simulink model "SHM_SIM"  (R2019b)
settings: Solver=ode23tb  StartTime=0.0  StopTime=T  MaxStep=1E-6  RelTol=1E-6
values from neighbouring files (symbols this model uses):
  f = 50    [SET_SIM.m]    (also in alphasolver.m = @(x) [(4/(pi))* VDC *(sin(x(1))-sin(x(2))+sin(x(3)))-V1)
  LL = 6.67e-3    (= 0.00667)    [SET_SIM.m]
  RL = 3.335    [SET_SIM.m]
  T_SMP = 2e-6    (= 2e-06)    [SET_SIM.m]
  VDC = 8.33    [SET_SIM.m]    (also in alphasolver.m = 24)
undefined symbols (not defined in the file or in its folder): a
libraries: powerlib x13, simulink x4, powerlib_meascontrol x2
settings Model: Creator=user  LastModifiedBy=ffara
settings DataIOCC: ReturnWorkspaceOutputs=off
settings DebuggingCC: ArithmeticOperatorsInVariantConditions=warning
settings SFSimCC: CustomCodeUndefinedFunction=UseInterfaceOnly

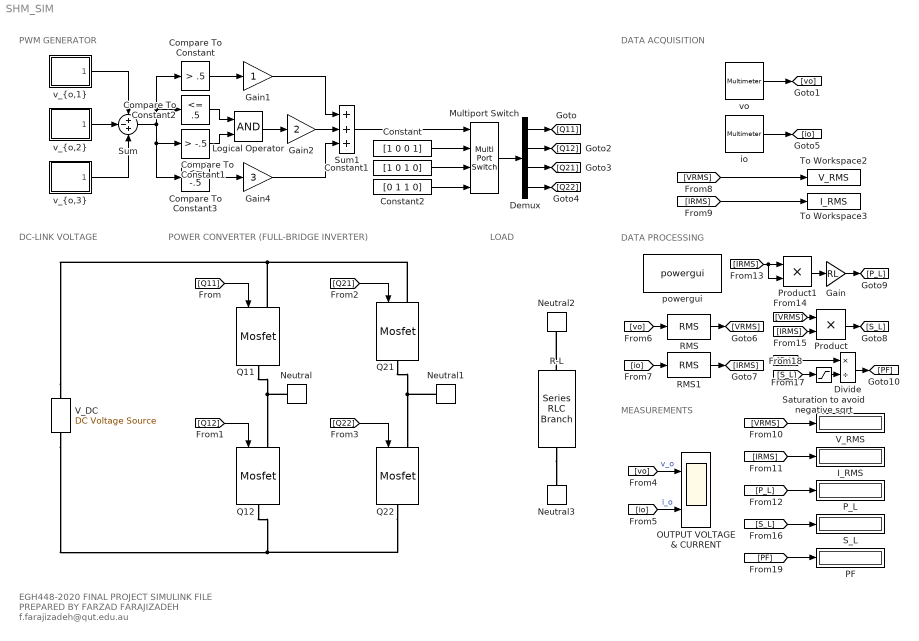
== system SHM_SIM ==
  note: EGH448-2020 FINAL PROJECT SIMULINK FILE
      | PREPARED BY FARZAD FARAJIZADEH
      | f.farajizadeh@qut.edu.au
  note: DATA ACQUISITION
  note: PWM GENERATOR
  note: LOAD
  note: POWER CONVERTER (FULL-BRIDGE INVERTER)
  note: DC-LINK VOLTAGE
  note: DATA PROCESSING
  note: MEASUREMENTS
  " OUTPUT VOLTAGE & CURRENT " : Scope  NumInputPorts=2
  Compare To Constant : simulink/Logic and Bit Operations/Compare To Constant  relop=>  const=.5  OutDataTypeStr=boolean
  Compare To Constant1 : simulink/Logic and Bit Operations/Compare To Constant  relop=>  const=-.5  OutDataTypeStr=boolean
  Compare To Constant2 : simulink/Logic and Bit Operations/Compare To Constant  relop=<=  const=.5  OutDataTypeStr=boolean
  Compare To Constant3 : simulink/Logic and Bit Operations/Compare To Constant  relop=<=  const=-.5  OutDataTypeStr=boolean
  Constant : Constant  Value=[1 0 0 1]
  Constant1 : Constant  Value=[1 0 1 0]
  Constant2 : Constant  Value=[0 1 1 0]
  Demux : Demux
  Divide : Product  Inputs=*/
  Gain : Gain  Gain=RL
  Gain1 : Gain
  Gain2 : Gain  Gain=2
  Gain4 : Gain  Gain=3
  I_RMS : Display
  Logical Operator : Logic  AllPortsSameDT=off  OutDataTypeStr=boolean
  Multiport Switch : MultiPortSwitch
  Neutral : powerlib/Elements/Neutral  LConnTagsString=a  NodeNumber=1
      settings: SourceProductName=Simscape Electrical  SourceProductBaseCode=PS
  Neutral1 : powerlib/Elements/Neutral  LConnTagsString=a  NodeNumber=2
      settings: SourceProductName=Simscape Electrical  SourceProductBaseCode=PS
  Neutral2 : powerlib/Elements/Neutral  LConnTagsString=a  NodeNumber=1
      settings: SourceProductName=Simscape Electrical  SourceProductBaseCode=PS
  Neutral3 : powerlib/Elements/Neutral  LConnTagsString=a  NodeNumber=2
      settings: SourceProductName=Simscape Electrical  SourceProductBaseCode=PS
  PF : Display
  P_L : Display
  Product : Product
  Product1 : Product
  Q{11..12,21..22} (4 alike) : powerlib/Power Electronics/Mosfet  Ron=0.001  Lon=0  Rd=0.001  Vfd=0  IC=0  Rs=1e5  Cs=inf  Measurements=off
      settings: SourceProductName=Simscape Electrical
  R-L : powerlib/Elements/Series RLC Branch  LConnTagsString=__new0  RConnTagsString=__new0  BranchType=RL  Resistance=RL  Inductance=LL  SetiL0=off  InitialCurrent=0  Capacitance=1e-6  Setx0=off  InitialVoltage=0  Measurements=Branch voltage and current
      settings: SourceProductName=Simscape Electrical
  RMS : powerlib_meascontrol/Measurements/RMS  TrueRMS=on  Freq=f  RMSInit=0  Ts=T_SMP
      settings: SourceProductName=Simscape Electrical
  RMS1 : powerlib_meascontrol/Measurements/RMS  TrueRMS=on  Freq=f  RMSInit=0  Ts=T_SMP
      settings: SourceProductName=Simscape Electrical
  S_L : Display
  Saturation to avoid negative sqrt : Saturate  UpperLimit=Inf  LowerLimit=1e-6  ZeroCross=off
  Sum : Sum  Inputs=+-+
  Sum1 : Sum  Inputs=+++
  To Workspace2 : ToWorkspace  VariableName=V_RMS  SampleTime=-1
      settings: MaxDataPoints=1
  To Workspace3 : ToWorkspace  VariableName=I_RMS  SampleTime=-1
      settings: MaxDataPoints=1
  V_DC : powerlib/Electrical Sources/DC Voltage Source  Amplitude=VDC  Measurements=None
      settings: SourceProductName=Simscape Electrical
  V_RMS : Display
  io : powerlib/Measurements/Multimeter  PhasorSimulation=off  OutputType=Complex  sel=2  L=2  Gain=1  yselected={'Ib: R-L'};  PSBOutputType=1  PSBequivalent=0  AxesSetting=[0,0.1,-100,100]  Display=0  SavedBlockNames=-11
      settings: SourceProductName=Simscape Electrical
  powergui : powerlib/powergui  Priority=1  SimulationMode=Discrete  SampleTime=T_SMP  frequency=60  Iterations=50  frequencyindice=0  Pbase=100e6  ErrMax=1e-4  UnitsV=kV  UnitsW=MW  buscounter=0  FunctionMessages=off  echomessages=off  EnableUseOfTLC=off  CurrentSourceSwitches=off  DisableSnubberDevices=off  DisableRonSwitches=off  DisableVfSwitches=off  DisplayEquations=off  AutomaticDiscreteSolvers=off  SolverType=Tustin/Backward Euler (TBE)  Interpol=off  ExternalGateDelay=off  methode=off  Ts=100  x0status=blocks  SPID=on  SwTol=0  HookPort=off  NonlinearTolerance=1e-4  nMaxIteration=100  ContinueOnMaxIteration=off  RestoreLinks=warning  ResistiveCurrentMeasurement=off  Frange=[0:2:500]  Ylog=off  Xlog=on  ShowGrid=off  save=off  variable=ZData  structure=VI_O  ZoomFFT=off  StartTime=0.0  cycles=20  DisplayStyle=3  fundamental=50  FreqAxis=off  MaxFrequency=800  frequencyindicesteady=1  RmsSteady=1  display=off
      settings: SourceProductName=Simscape Electrical
  "v_{o,1}" : Subsystem  mask{a=a(1)}
      mask prompts: a "Angle Shift (Deg):"
      mask DialogControl DescGroupVar Prompt: Angle Shift
  "v_{o,2}" : Subsystem  mask{a=a(2)}
      mask prompts: a "Angle Shift (Deg):"
      mask DialogControl DescGroupVar Prompt: Angle Shift
  "v_{o,3}" : Subsystem  mask{a=a(3)}
      mask prompts: a "Angle Shift (Deg):"
      mask DialogControl DescGroupVar Prompt: Angle Shift
  vo : powerlib/Measurements/Multimeter  PhasorSimulation=off  OutputType=Complex  sel=1  L=2  Gain=1  yselected={'Ub: R-L'};  PSBOutputType=1  PSBequivalent=0  AxesSetting=[0,0.1,-100,100]  Display=0  SavedBlockNames=-11
      settings: SourceProductName=Simscape Electrical
  wires:
  "v_{o,1}"/1("v_{o,i}") -> Sum/1
  "v_{o,3}"/1("v_{o,i}") -> Sum/3
  "v_{o,2}"/1("v_{o,i}") -> Sum/2
  Sum/1 -> Compare To Constant3/1, Compare To Constant1/1, Compare To Constant/1, Compare To Constant2/1
  Compare To Constant/1 -> Gain1/1
  Compare To Constant2/1 -> Logical Operator/1
  Compare To Constant1/1 -> Logical Operator/2
  Compare To Constant3/1 -> Gain4/1
  Logical Operator/1 -> Gain2/1
  Gain1/1 -> Sum1/1
  Gain2/1 -> Sum1/2
  Gain4/1 -> Sum1/3
  Sum1/1 -> Multiport Switch/1
  Constant/1 -> Multiport Switch/2
  Constant1/1 -> Multiport Switch/3
  Constant2/1 -> Multiport Switch/4
  Multiport Switch/1 -> Demux/1
  Demux/1 -> [Q11]
  Demux/2 -> [Q12]
  Demux/3 -> [Q21]
  Demux/4 -> [Q22]
  [Q11] -> Q11/1
  [Q12] -> Q12/1
  [Q21] -> Q21/1
  [Q22] -> Q22/1
  vo/1 -> [vo]
  [vo] -> " OUTPUT VOLTAGE & CURRENT "/1  "v_o"
  io/1 -> [io]
  [io] -> " OUTPUT VOLTAGE & CURRENT "/2  "i_o"
  [vo] -> RMS/1
  [io] -> RMS1/1
  RMS/1 -> [VRMS]
  RMS1/1 -> [IRMS]
  [VRMS] -> To Workspace2/1
  [IRMS] -> To Workspace3/1
  [VRMS] -> V_RMS/1
  [IRMS] -> I_RMS/1
  [IRMS] -> Product/2
  [VRMS] -> Product/1
  Product/1 -> [S_L]
  Product1/1 -> Gain/1
  [IRMS] -> Product1/2, Product1/1
  Gain/1 -> [P_L]
  [S_L] -> S_L/1
  [P_L] -> P_L/1
  [P_L] -> Divide/1
  [S_L] -> Saturation to avoid negative sqrt/1
  [PF] -> PF/1
  Divide/1 -> [PF]
  Saturation to avoid negative sqrt/1 -> Divide/2
  connections:
  Q11/RConn1 -- Neutral/LConn1 -- Q12/LConn1
  V_DC/RConn1 -- Q11/LConn1 -- Q21/LConn1
  V_DC/LConn1 -- Q12/RConn1 -- Q22/RConn1
  Q21/RConn1 -- Neutral1/LConn1 -- Q22/LConn1
  R-L/LConn1 -- Neutral2/LConn1
  R-L/RConn1 -- Neutral3/LConn1

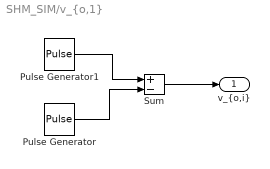
== system SHM_SIM/v_{o,1} ==
  Pulse Generator : DiscretePulseGenerator  PulseType=Time based  Period=1/f  PulseWidth=50  PhaseDelay=(.5/f)*a*(1/180)
  Pulse Generator1 : DiscretePulseGenerator  PulseType=Time based  Period=1/f  PulseWidth=50  PhaseDelay=-(.5/f)*a*(1/180)
  Sum : Sum  Inputs=+-
  "v_{o,i}" : Outport  VectorParamsAs1DForOutWhenUnconnected=off
  wires:
  Pulse Generator1/1 -> Sum/1
  Sum/1 -> "v_{o,i}"/1
  Pulse Generator/1 -> Sum/2

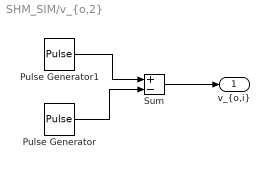
== system SHM_SIM/v_{o,2} ==
  Pulse Generator : DiscretePulseGenerator  PulseType=Time based  Period=1/f  PulseWidth=50  PhaseDelay=(.5/f)*a*(1/180)
  Pulse Generator1 : DiscretePulseGenerator  PulseType=Time based  Period=1/f  PulseWidth=50  PhaseDelay=-(.5/f)*a*(1/180)
  Sum : Sum  Inputs=+-
  "v_{o,i}" : Outport  VectorParamsAs1DForOutWhenUnconnected=off
  wires:
  Pulse Generator/1 -> Sum/2
  Sum/1 -> "v_{o,i}"/1
  Pulse Generator1/1 -> Sum/1

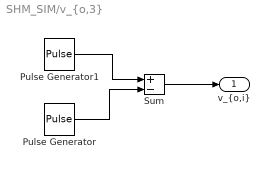
== system SHM_SIM/v_{o,3} ==
  Pulse Generator : DiscretePulseGenerator  PulseType=Time based  Period=1/f  PulseWidth=50  PhaseDelay=(.5/f)*a*(1/180)
  Pulse Generator1 : DiscretePulseGenerator  PulseType=Time based  Period=1/f  PulseWidth=50  PhaseDelay=-(.5/f)*a*(1/180)
  Sum : Sum  Inputs=+-
  "v_{o,i}" : Outport  VectorParamsAs1DForOutWhenUnconnected=off
  wires:
  Pulse Generator1/1 -> Sum/1
  Sum/1 -> "v_{o,i}"/1
  Pulse Generator/1 -> Sum/2
